simulink model "BattEv_Simscape"  (R2023a)
settings: Solver=ode23t  StartTime=0  StopTime=inf  RelTol=1e-3  EnableMultiTasking=on
model workspace (MAT data in the model file):
  Active_Scenario_Index = 1
  BattCurrent = [0 0.1 0.2 0.3 0.4 0.5 0.6 0.7 0.8 0.9 1 1.1 ... (49482 elements, 24741x2)]
  BattSocInit = 0.75
  BattTempInit = 25
  Battery : object (value not decoded)
  CellType = 1
  EV_current = 200
  EV_motion = [20 4 0.8]
  EV_sf = 2000
  Fs = 0
  Fv = 0.0025
  Jcomp = 0.0227
  Ki = 251.3274
  Kisa = 346.6583
  Kp_d = 0.47149
  Kp_q = 0.52125
  Ksa = 85.4316
  Ksf = 1996.2651
  Ld = 0.0003752
  Ldq = [0.0003752 0.0004148]
  Lq = 0.0004148
  Mechanical = [0.0227 0.0025 0]
  Np_Module = 31
  Ns_Module = 24
  NumModules = 4
  OverCellVoltageLimit = 4.19999980927
  P = 4
  PolePairs = 4
  R_bleed = 20
  Rs = 0.2
  T_eff_bp = [0 32.1428571429 64.2857142857 96.4285714286 128.571428571 160.714285714 192.857142857 225 257.142857143 289.285714286 321.428571429 353.571428571 ... (15 elements, 1x15)]
  T_env = 30
  T_init = 303.15
  T_max = 450
  T_mtpa = [0 13.3131834767 26.6278836885 39.9456159322 53.2678926341 66.5962219318 79.9321062746 93.277041051 106.632513247 120.000000141]
  T_set = 20.5
  Tc = 0.02
  TempInit = 288.15
  TestCase = 1
  UnderCellVoltageLimit = 2.5
  ba = 3.4029
  cell_area = 0.101908
  efficiency_table = [86.7 86.7 86.7 86.7 86.7 86.7 86.7 86.7 86.7 86.7 86.7 86.7 ... (180 elements, 12x15)]
  h_conv = 5
  id_mtpa = [0 -0.114523352646 -0.457989076459 -1.03008464374 -1.83029075221 -2.85788367342 -4.11193850568 -5.59133329791 -7.29475400168 -9.22070020138]
  idq0 = [0 0]
  idq_limits = [-9.220699542 166.993501392 167.247872355]
  iq_mtpa = [0 18.5827440345 37.1633719111 55.7397734896 74.3098506185 92.871523015 111.422734008 129.961456105 148.485696337 166.993501356]
  lambda_pm = 0.1194
  losses_table = [0 0 0 0 0 0 0 0 0 0 0 0 ... (180 elements, 12x15)]
  mdot_rev = 0.01
  mechanical = [0.0227 0.0025 0]
  omega_init = 0
  pipe : object (value not decoded)
  power_max = 211000
  pump : object (value not decoded)
  radiator : object (value not decoded)
  t_sim = 2474
  tank : object (value not decoded)
  theta_init = 0
  torque_max = 450
  ts = 0.1
  valve : object (value not decoded)
  w_eff_bp = [0 1600 3200 4477.56 4800 6400 8000 9600 11200 12800 14400 16000]
libraries: autolibpowerinfoutils x10, fl_lib x7, nesl_utility_internal x6, ee_lib x1
(part 2 of 2)

== system BattEv_Simscape/Battery Power Accounting ==
  BattV : Inport
  BattCurr : Inport  Port=2
  Bus Creator : BusCreator  Inputs=1
  Bus Creator1 : BusCreator  Inputs=1
  Gain : Gain  Gain=-1
  Gain1 : Gain
  Power Accounting : autolibpowerinfoutils/Power Accounting Bus Creator  AssctBlkSelPopup=Parent  RefBlkName='autolibsharedcoupling/Torsional Compliance'  PwrTrnsfrdCheckBox=on  PwrNotTrnsfrdCheckBox=on  PwrStoredCheckBox=off  aMode=aMode
  Product3 : Product
  Terminator2 : Terminator
  wires:
  Bus Creator/1 -> Power Accounting/1  "PwrTranfred"
  Gain/1 -> Bus Creator/1  "Batttransferred"
  Power Accounting/1 -> Terminator2/1
  Gain1/1 -> Bus Creator1/1  "BattNotTransferd"
  BattV/1 -> Product3/1
  BattCurr/1 -> Product3/2
  Bus Creator1/1 -> Power Accounting/2  "PwrNotTranfred"
  Product3/1 -> Gain1/1, Gain/1  "BattPwr"

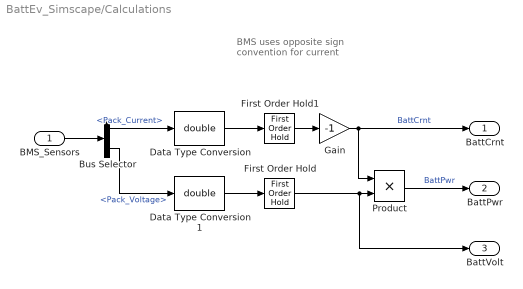
== system BattEv_Simscape/Calculations ==
  note: BMS uses opposite
      | sign convention for
      | current
  BMS_Sensors : Inport
  Bus Selector : BusSelector  OutputSignals=Pack_Current,Pack_Voltage
  Data Type Conversion : DataTypeConversion  OutDataTypeStr=double  SaturateOnIntegerOverflow=off  RndMeth=Floor
  Data Type Conversion1 : DataTypeConversion  OutDataTypeStr=double  SaturateOnIntegerOverflow=off  RndMeth=Floor
  First Order Hold : FirstOrderHold  ErrorTolerance=inf  AllowContinuousInput=on
  First Order Hold1 : FirstOrderHold  ErrorTolerance=inf  AllowContinuousInput=on
  Gain : Gain  Gain=-1
  Product : Product
  BattCrnt : Outport
  BattPwr : Outport  Port=2
  BattVolt : Outport  Port=3
  wires:
  Gain/1 -> BattCrnt/1, Product/1  "BattCrnt"
  BMS_Sensors/1 -> Bus Selector/1
  Data Type Conversion/1 -> First Order Hold1/1
  First Order Hold/1 -> BattVolt/1, Product/2
  First Order Hold1/1 -> Gain/1
  Bus Selector/1 -> Data Type Conversion/1  "<Pack_Current>"
  Bus Selector/2 -> Data Type Conversion1/1  "<Pack_Voltage>"
  Data Type Conversion1/1 -> First Order Hold/1
  Product/1 -> BattPwr/1  "BattPwr"

== system BattEv_Simscape/Cooling System ==
  BMS_Sensors : Inport
  AmbTmp : Inport  Port=2
  VehSpd : Inport  Port=3
  "Simscape " : Subsystem  VariantControl=1  ReferencedSubsystem=sscfluids_ev_battery_cooling_variant
      settings: PortSchema="{\"entries\":[{\"content\":{\"sides\":[{\"content\":{\"connectorIds\":[\"In1\",\"LConn1\",\"LConn2\",\"LConn3\",\"LConn4\",\"In3\",\"In2\"]},\"type\":\"ConnectorPlacement.EquallySpacedRectSide\",\"uuid\":\"91345e43-9326-4851-ae22-0115818e13bd\"},{\"content\":{\"connectorIds\":[\"RConn1\"],\"side\":\"RIGHT\"},\"type\":\"ConnectorPlacement.EquallySpacedRectSide\",\"uuid\":\"8fdec940-c4a1-4379-aa74-e54f16fb1812\"},{\"content\":{\"side\":\"TOP\"},\"type\":\"ConnectorPlacement.EquallySpacedRectSide\",\"uuid\":\"514fe1d2-faac-427c-8664-9f81e8916636\"}]},\"type\":\"ConnectorPlacement.EquallySpacedConnector\",\"uuid\":\"a4d1e3fd-26b0-4676-91d7-dc7f8f7b5942\"}],\"packageUris\":[\"http://schema.mathworks.com/mf0/Connector/R2020b\"],\"version\":\"1.0\"}"
  Pack 4 : PMIOPort  Side=Left
  Pack 3 : PMIOPort  Port=2  Side=Left
  Pack 2 : PMIOPort  Port=3  Side=Left
  Pack 1 : PMIOPort  Port=4  Side=Left
  Mot_H : PMIOPort  Port=5  Side=Right

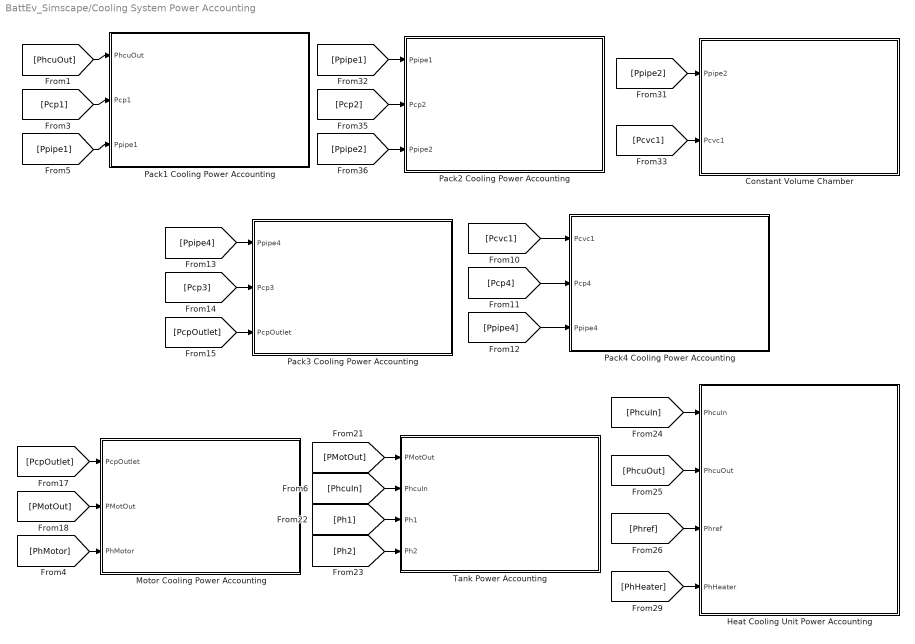
== system BattEv_Simscape/Cooling System Power Accounting ==
  Constant Volume Chamber : Subsystem
  Heat Cooling Unit Power Accounting : Subsystem
  Motor Cooling Power Accounting : Subsystem
  Pack1 Cooling Power Accounting : Subsystem
  Pack2 Cooling Power Accounting : Subsystem
  Pack3 Cooling Power Accounting : Subsystem
  Pack4 Cooling Power Accounting : Subsystem
  Tank Power Accounting : Subsystem
  wires:
  [Ph2] -> Tank Power Accounting/4(Ph2)
  [Ppipe2] -> Pack2 Cooling Power Accounting/3(Ppipe2)
  [Pcp2] -> Pack2 Cooling Power Accounting/2(Pcp2)
  [Phref] -> Heat Cooling Unit Power Accounting/3(Phref)
  [PMotOut] -> Motor Cooling Power Accounting/2(PMotOut)
  [PhcuIn] -> Tank Power Accounting/2(PhcuIn)
  [PcpOutlet] -> Motor Cooling Power Accounting/1(PcpOutlet)
  [PhcuIn] -> Heat Cooling Unit Power Accounting/1(PhcuIn)
  [PhcuOut] -> Pack1 Cooling Power Accounting/1(PhcuOut)
  [PhcuOut] -> Heat Cooling Unit Power Accounting/2(PhcuOut)
  [PcpOutlet] -> Pack3 Cooling Power Accounting/3(PcpOutlet)
  [Ppipe1] -> Pack1 Cooling Power Accounting/3(Ppipe1)
  [Pcp1] -> Pack1 Cooling Power Accounting/2(Pcp1)
  [Pcp3] -> Pack3 Cooling Power Accounting/2(Pcp3)
  [Pcvc1] -> Constant Volume Chamber/2(Pcvc1)
  [Ppipe4] -> Pack3 Cooling Power Accounting/1(Ppipe4)
  [Pcvc1] -> Pack4 Cooling Power Accounting/1(Pcvc1)
  [Ppipe1] -> Pack2 Cooling Power Accounting/1(Ppipe1)
  [Ppipe4] -> Pack4 Cooling Power Accounting/3(Ppipe4)
  [Ph1] -> Tank Power Accounting/3(Ph1)
  [PhMotor] -> Motor Cooling Power Accounting/3(PhMotor)
  [Ppipe2] -> Constant Volume Chamber/1(Ppipe2)
  [PMotOut] -> Tank Power Accounting/1(PMotOut)
  [PhHeater] -> Heat Cooling Unit Power Accounting/4(PhHeater)
  [Pcp4] -> Pack4 Cooling Power Accounting/2(Pcp4)

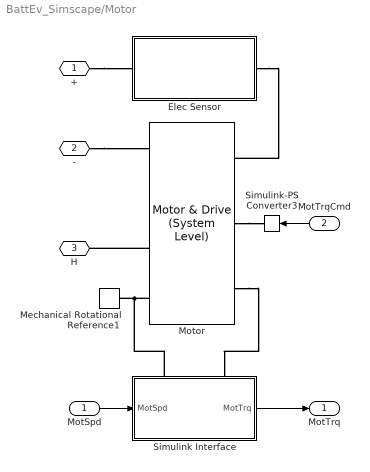
== system BattEv_Simscape/Motor ==
  MotSpd : Inport
  MotTrqCmd : Inport  Port=2
  Elec Sensor : Subsystem
  Mechanical Rotational Reference1 : fl_lib/Mechanical/Rotational Elements/Mechanical Rotational Reference
  Motor : ee_lib/Electromechanical/Motor & Drive (System Level)  torque_speed_param=ee.enum.electromech.envelope.torque_power  overtorque_param=ee.enum.electromech.overtorque.no  T_t=torque_max N*m  T_t_intermittent=[.36, .32, .28, 0] N*m  T_t_2D=[.09, .09, .09; .08, .08, .08; .07, .07, .07; 0, 0, 0] N*m  T_t_intermittent_2D=[.36, .36, .36; .32, .32, .32; .28, .28, .28; 0, 0, 0] N*m  w_t=Mot.w_eff_bp_EV_rear rpm  vdc_t=[6, 12, 24] V  torque_max=torque_max N*m  power_max=power_max W  torque_max_intermittent=0.4 N*m  power_max_intermittent=120 W  time_overtorque=30 s  time_recover=60 s  Tc=Tc s  losses_param=3  eff=100  w_eff=3750 rpm  T_eff=0.08 N*m  Piron=0 W  Pbase=0 W  w_eff_vec=w_eff_bp.*pi/30 rad/s  T_eff_vec=T_eff_bp N*m  v_eff_vec=[100, 250, 400] V  losses_mat=[1.49, 1.67, 2.21, 3.1; .42, .69, 1.14, 2.03; .06, .24, .78, 1.68; .42, .69, 1.14, 2.03; 1.49, 1.67, 2.21, 3.1] W  efficiency_mat=efficiency_table  losses_mat_3D=ones(5, 4, 3) W  efficiency_mat_3D=95 * ones(5, 4, 3)  Res=0 %Mot.supplyRes Ohm  enable_fault=simscape.enum.onoff.off  fault_condition=1  fault_threshold=0.5  J=5e-6 %Mot.inertia kg*m^2  lam=0 %Mot.damping N*m/(rad/s)  speed0=0 rpm  faulted_specify=off  faulted_priority=None  faulted=0  faulted_nominal_specify=off  faulted_nominal_unit=1  faulted_nominal_value=1  torqueLimitContinuous_specify=off  torqueLimitContinuous_priority=None  torqueLimitContinuous=0 N*m  torqueLimitContinuous_nominal_specify=off  torqueLimitContinuous_nominal_unit=N*m  torqueLimitContinuous_nominal_value=1  alpha=3.93e-3 1/K  Tmeas=25 degC  Tmeas2=125 degC  losses_mat_T2=[1.49, 1.74, 2.49, 3.74; .42, .67, 1.42, 2.67; .06, .31, 1.06, 2.31; .42, .67, 1.42, 2.67; 1.49, 1.74, 2.49, 3.74] W  efficiency_mat_T2=efficiency_table  losses_mat_3D_T2=ones(5, 4, 3) W  efficiency_mat_3D_T2=95 * ones(5, 4, 3)  thermal_mass=800 %Mot.thermalMass J/K  initial_temperature=300 K
      settings: InternalSimscapePortConfiguration="{\"Bottom\":[],\"Left\":[{\"id\":\"Vp\",\"label\":\"+\",\"type\":\"foundation.electrical.electrical\"},{\"id\":\"Tr\",\"label\":\"Tr\",\"type\":\"input\"},{\"id\":\"R\",\"label\":\"R\",\"type\":\"foundation.mechanical.rotational.rotational\"}],\"Right\":[{\"id\":\"Vm\",\"label\":\"-\",\"type\":\"foundation.electrical.electrical\"},{\"id\":\"Omega\",\"label\":\"w\",\"type\":\"output\"},{\"id\":\"H\",\"label\":\"H\",\"type\":\"foundation.thermal.thermal\"},{\"id\":\"C\",\"label\":\"C\",\"type\":\"foundation.mechanical.rotational.rotational\"}],\"Top\":[]}"
  Simulink Interface : Subsystem
      settings: PortSchema="{\"entries\":[{\"content\":{\"sides\":[{\"content\":{\"connectorIds\":[\"In1\"]},\"type\":\"ConnectorPlacement.EquallySpacedRectSide\",\"uuid\":\"bf4125d2-d804-43ee-b309-19af55b24a20\"},{\"content\":{\"connectorIds\":[\"Out1\"],\"side\":\"RIGHT\"},\"type\":\"ConnectorPlacement.EquallySpacedRectSide\",\"uuid\":\"b387e632-ddea-4493-9ae8-5e997efec9a6\"},{\"content\":{\"connectorIds\":[\"LConn1\",\"LConn2\"],\"side\":\"TOP\"},\"type\":\"ConnectorPlacement.EquallySpacedRectSide\",\"uuid\":\"41fd5ea6-0488-466e-8be0-697a42498d14\"}]},\"type\":\"ConnectorPlacement.EquallySpacedConnector\",\"uuid\":\"25cf6a75-933f-4ef5-8c77-b93f7c2ffe1f\"}],\"packageUris\":[\"http://schema.mathworks.com/mf0/Connector/R2020b\"],\"version\":\"1.0\"}"
  Simulink-PS Converter3 : nesl_utility_internal/Simulink-PS Converter  PhysicalDomain=network_engine_domain  SubClassName=ps_input  LeftPortType=input  RightPortType=output  PseudoPeriodic=off  Frequencies=[]  NoiseDistribution=none  NoiseParameters=[]  Unit=N*m  AffineConversion=off  FilteringAndDerivatives=provide  SimscapeFilterOrder=1  InputFilterTimeConstant=0.001  UdotUserProvided=0
  + : PMIOPort  Side=Left
  - : PMIOPort  Port=2  Side=Left
  H : PMIOPort  Port=3  Side=Left
  MotTrq : Outport  VectorParamsAs1DForOutWhenUnconnected=off
  wires:
  MotSpd/1 -> Simulink Interface/1(MotSpd)
  Simulink Interface/1(MotTrq) -> MotTrq/1
  MotTrqCmd/1 -> Simulink-PS Converter3/1
  connections:
  -/RConn1 -- Motor/RConn1
  Simulink Interface/LConn1 -- Motor/RConn4 -- Mechanical Rotational Reference1/LConn1
  Motor/LConn2 -- Simulink-PS Converter3/RConn1
  Motor/LConn3 -- Simulink Interface/LConn2
  +/RConn1 -- Elec Sensor/LConn1
  Elec Sensor/RConn1 -- Motor/LConn1
  Motor/RConn3 -- H/RConn1

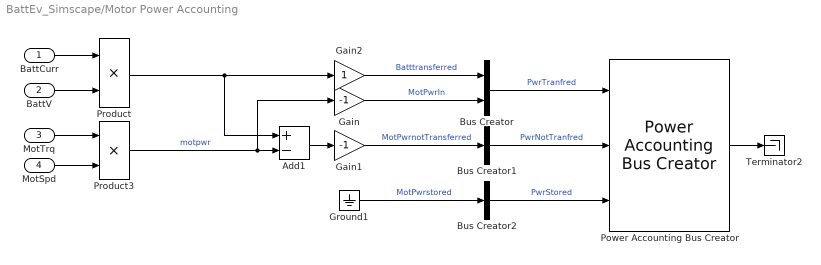
== system BattEv_Simscape/Motor Power Accounting ==
  BattCurr : Inport
  BattV : Inport  Port=2
  MotTrq : Inport  Port=3
  MotSpd : Inport  Port=4
  Add1 : Sum  Inputs=+-
  Bus Creator : BusCreator  Inputs=2
  Bus Creator1 : BusCreator  Inputs=1
  Bus Creator2 : BusCreator  Inputs=1
  Gain : Gain  Gain=-1
  Gain1 : Gain  Gain=-1
  Gain2 : Gain
  Ground1 : Ground
  Power Accounting Bus Creator : autolibpowerinfoutils/Power Accounting Bus Creator  AssctBlkSelPopup=Parent  RefBlkName='autolibsharedcoupling/Torsional Compliance'  PwrTrnsfrdCheckBox=on  PwrNotTrnsfrdCheckBox=on  PwrStoredCheckBox=on  aMode=aMode
  Product : Product
  Product3 : Product
  Terminator2 : Terminator
  wires:
  Gain2/1 -> Bus Creator/1  "Batttransferred"
  Product/1 -> Add1/1, Gain2/1
  BattV/1 -> Product/2
  BattCurr/1 -> Product/1
  Bus Creator/1 -> Power Accounting Bus Creator/1  "PwrTranfred"
  Gain/1 -> Bus Creator/2  "MotPwrIn"
  Power Accounting Bus Creator/1 -> Terminator2/1
  Ground1/1 -> Bus Creator2/1  "MotPwrstored"
  MotTrq/1 -> Product3/1
  MotSpd/1 -> Product3/2
  Bus Creator1/1 -> Power Accounting Bus Creator/2  "PwrNotTranfred"
  Bus Creator2/1 -> Power Accounting Bus Creator/3  "PwrStored"
  Product3/1 -> Gain/1, Add1/2  "motpwr"
  Gain1/1 -> Bus Creator1/1  "MotPwrnotTransferred"
  Add1/1 -> Gain1/1

== system BattEv_Simscape/Subsystem2 ==
  In Bus Element : Inport  PortName=BMS_Info  Element=SOC
  Bus Selector : BusSelector  OutputSignals=SOC_CC
  Data Type Conversion : DataTypeConversion  SaturateOnIntegerOverflow=off  RndMeth=Floor
  Rate Transition : RateTransition  Commented=through
  convert2percent : Gain  Gain=100
  BattSOC : Outport
  wires:
  In Bus Element/1 -> Bus Selector/1
  convert2percent/1 -> Data Type Conversion/1
  Bus Selector/1 -> convert2percent/1  "<SOC_CC>"
  Data Type Conversion/1 -> Rate Transition/1
  Rate Transition/1 -> BattSOC/1

== system BattEv_Simscape/Cooling System Power Accounting/Constant Volume Chamber ==
  Ppipe2 : Inport
  Pcvc1 : Inport  Port=2
  " Power Accounting" : autolibpowerinfoutils/Power Accounting Bus Creator  AssctBlkSelPopup=Parent  RefBlkName='autolibsharedcoupling/Torsional Compliance'  PwrTrnsfrdCheckBox=on  PwrNotTrnsfrdCheckBox=on  PwrStoredCheckBox=off  aMode=aMode
  Add : Sum  Inputs=+-
  Bus Creator : BusCreator  Inputs=2
  Bus Creator1 : BusCreator  Inputs=1
  Gain : Gain  Gain=-1
  Gain1 : Gain  Gain=-1
  Terminator2 : Terminator
  wires:
  Ppipe2/1 -> Bus Creator/1, Add/1  "Ppipe2"
  Gain/1 -> Bus Creator/2  "Pcvc1"
  Bus Creator/1 -> " Power Accounting"/1  "PwrTranfred"
  Pcvc1/1 -> Add/2, Gain/1
  Gain1/1 -> Bus Creator1/1  "PwrNotTrnsfrd"
  Bus Creator1/1 -> " Power Accounting"/2  "PwrNotTranfred"
  " Power Accounting"/1 -> Terminator2/1
  Add/1 -> Gain1/1

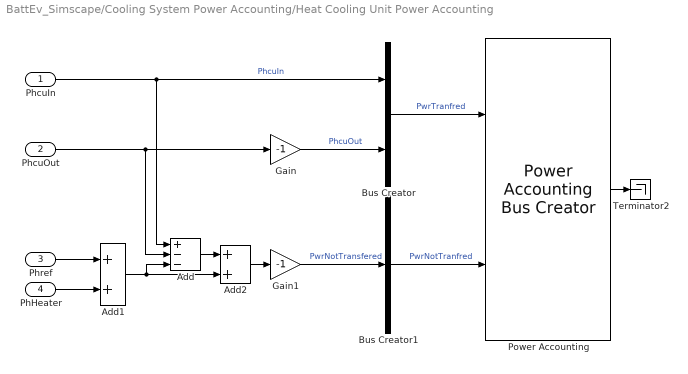
== system BattEv_Simscape/Cooling System Power Accounting/Heat Cooling Unit Power Accounting ==
  PhcuIn : Inport
  PhcuOut : Inport  Port=2
  Phref : Inport  Port=3
  PhHeater : Inport  Port=4
  Add : Sum  Inputs=+--
  Add1 : Sum
  Add2 : Sum
  Bus Creator : BusCreator  Inputs=2
  Bus Creator1 : BusCreator  Inputs=1
  Gain : Gain  Gain=-1
  Gain1 : Gain  Gain=-1
  Power Accounting : autolibpowerinfoutils/Power Accounting Bus Creator  AssctBlkSelPopup=Parent  RefBlkName='autolibsharedcoupling/Torsional Compliance'  PwrTrnsfrdCheckBox=on  PwrNotTrnsfrdCheckBox=on  PwrStoredCheckBox=off  aMode=aMode
  Terminator2 : Terminator
  wires:
  PhcuOut/1 -> Add/2, Gain/1
  Add2/1 -> Gain1/1
  Power Accounting/1 -> Terminator2/1
  Bus Creator1/1 -> Power Accounting/2  "PwrNotTranfred"
  Phref/1 -> Add1/1
  Gain1/1 -> Bus Creator1/1  "PwrNotTransfered"
  Bus Creator/1 -> Power Accounting/1  "PwrTranfred"
  Gain/1 -> Bus Creator/2  "PhcuOut"
  PhcuIn/1 -> Bus Creator/1, Add/1  "PhcuIn"
  PhHeater/1 -> Add1/2
  Add1/1 -> Add/3, Add2/2
  Add/1 -> Add2/1

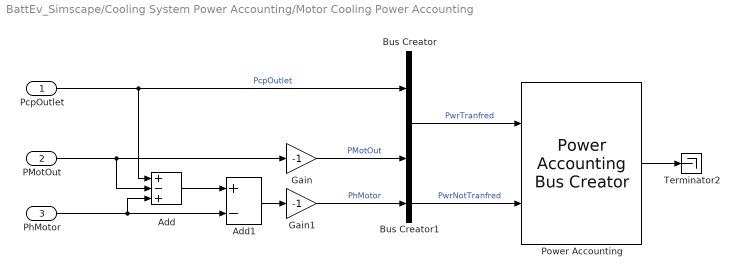
== system BattEv_Simscape/Cooling System Power Accounting/Motor Cooling Power Accounting ==
  PcpOutlet : Inport
  PMotOut : Inport  Port=2
  PhMotor : Inport  Port=3
  Add : Sum  Inputs=+-+
  Add1 : Sum  Inputs=+-
  Bus Creator : BusCreator  Inputs=2
  Bus Creator1 : BusCreator  Inputs=1
  Gain : Gain  Gain=-1
  Gain1 : Gain  Gain=-1
  Power Accounting : autolibpowerinfoutils/Power Accounting Bus Creator  AssctBlkSelPopup=Parent  RefBlkName='autolibsharedcoupling/Torsional Compliance'  PwrTrnsfrdCheckBox=on  PwrNotTrnsfrdCheckBox=on  PwrStoredCheckBox=off  aMode=aMode
  Terminator2 : Terminator
  wires:
  Add1/1 -> Gain1/1
  Power Accounting/1 -> Terminator2/1
  Bus Creator1/1 -> Power Accounting/2  "PwrNotTranfred"
  Add/1 -> Add1/1
  Gain1/1 -> Bus Creator1/1  "PhMotor"
  PMotOut/1 -> Gain/1, Add/2
  Bus Creator/1 -> Power Accounting/1  "PwrTranfred"
  Gain/1 -> Bus Creator/2  "PMotOut"
  PcpOutlet/1 -> Bus Creator/1, Add/1  "PcpOutlet"
  PhMotor/1 -> Add1/2, Add/3

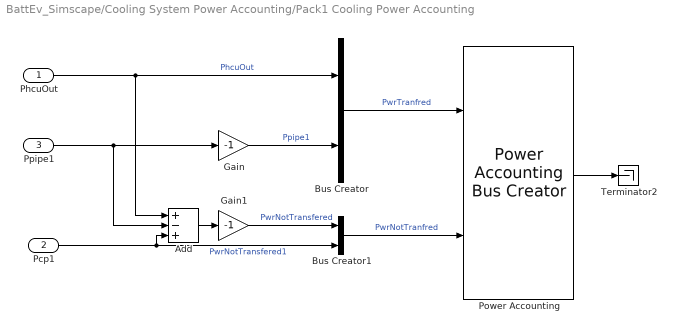
== system BattEv_Simscape/Cooling System Power Accounting/Pack1 Cooling Power Accounting ==
  PhcuOut : Inport
  Pcp1 : Inport  Port=2
  Ppipe1 : Inport  Port=3
  Add : Sum  Inputs=+-+
  Bus Creator : BusCreator  Inputs=2
  Bus Creator1 : BusCreator  Inputs=2
  Gain : Gain  Gain=-1
  Gain1 : Gain  Gain=-1
  Power Accounting : autolibpowerinfoutils/Power Accounting Bus Creator  AssctBlkSelPopup=Parent  RefBlkName='autolibsharedcoupling/Torsional Compliance'  PwrTrnsfrdCheckBox=on  PwrNotTrnsfrdCheckBox=on  PwrStoredCheckBox=off  aMode=aMode
  Terminator2 : Terminator
  wires:
  Add/1 -> Gain1/1
  Power Accounting/1 -> Terminator2/1
  Bus Creator1/1 -> Power Accounting/2  "PwrNotTranfred"
  Gain1/1 -> Bus Creator1/1  "PwrNotTransfered"
  Ppipe1/1 -> Gain/1, Add/2
  Bus Creator/1 -> Power Accounting/1  "PwrTranfred"
  Gain/1 -> Bus Creator/2  "Ppipe1"
  PhcuOut/1 -> Bus Creator/1, Add/1  "PhcuOut"
  Pcp1/1 -> Add/3, Bus Creator1/2  "PwrNotTransfered1"

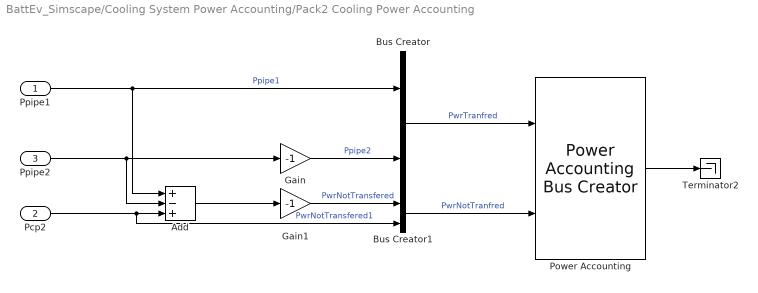
== system BattEv_Simscape/Cooling System Power Accounting/Pack2 Cooling Power Accounting ==
  Ppipe1 : Inport
  Pcp2 : Inport  Port=2
  Ppipe2 : Inport  Port=3
  Add : Sum  Inputs=+-+
  Bus Creator : BusCreator  Inputs=2
  Bus Creator1 : BusCreator  Inputs=2
  Gain : Gain  Gain=-1
  Gain1 : Gain  Gain=-1
  Power Accounting : autolibpowerinfoutils/Power Accounting Bus Creator  AssctBlkSelPopup=Parent  RefBlkName='autolibsharedcoupling/Torsional Compliance'  PwrTrnsfrdCheckBox=on  PwrNotTrnsfrdCheckBox=on  PwrStoredCheckBox=off  aMode=aMode
  Terminator2 : Terminator
  wires:
  Pcp2/1 -> Bus Creator1/2, Add/3  "PwrNotTransfered1"
  Ppipe1/1 -> Bus Creator/1, Add/1  "Ppipe1"
  Gain/1 -> Bus Creator/2  "Ppipe2"
  Bus Creator/1 -> Power Accounting/1  "PwrTranfred"
  Ppipe2/1 -> Add/2, Gain/1
  Gain1/1 -> Bus Creator1/1  "PwrNotTransfered"
  Bus Creator1/1 -> Power Accounting/2  "PwrNotTranfred"
  Power Accounting/1 -> Terminator2/1
  Add/1 -> Gain1/1

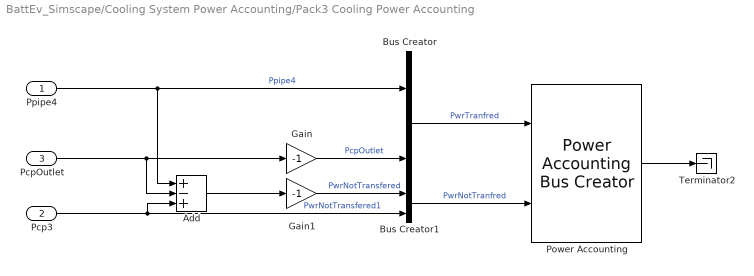
== system BattEv_Simscape/Cooling System Power Accounting/Pack3 Cooling Power Accounting ==
  Ppipe4 : Inport
  Pcp3 : Inport  Port=2
  PcpOutlet : Inport  Port=3
  Add : Sum  Inputs=+-+
  Bus Creator : BusCreator  Inputs=2
  Bus Creator1 : BusCreator  Inputs=2
  Gain : Gain  Gain=-1
  Gain1 : Gain  Gain=-1
  Power Accounting : autolibpowerinfoutils/Power Accounting Bus Creator  AssctBlkSelPopup=Parent  RefBlkName='autolibsharedcoupling/Torsional Compliance'  PwrTrnsfrdCheckBox=on  PwrNotTrnsfrdCheckBox=on  PwrStoredCheckBox=off  aMode=aMode
  Terminator2 : Terminator
  wires:
  Pcp3/1 -> Bus Creator1/2, Add/3  "PwrNotTransfered1"
  Ppipe4/1 -> Bus Creator/1, Add/1  "Ppipe4"
  Gain/1 -> Bus Creator/2  "PcpOutlet"
  Bus Creator/1 -> Power Accounting/1  "PwrTranfred"
  PcpOutlet/1 -> Add/2, Gain/1
  Gain1/1 -> Bus Creator1/1  "PwrNotTransfered"
  Bus Creator1/1 -> Power Accounting/2  "PwrNotTranfred"
  Power Accounting/1 -> Terminator2/1
  Add/1 -> Gain1/1

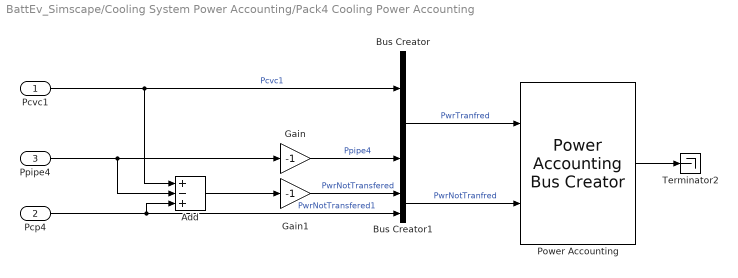
== system BattEv_Simscape/Cooling System Power Accounting/Pack4 Cooling Power Accounting ==
  Pcvc1 : Inport
  Pcp4 : Inport  Port=2
  Ppipe4 : Inport  Port=3
  Add : Sum  Inputs=+-+
  Bus Creator : BusCreator  Inputs=2
  Bus Creator1 : BusCreator  Inputs=2
  Gain : Gain  Gain=-1
  Gain1 : Gain  Gain=-1
  Power Accounting : autolibpowerinfoutils/Power Accounting Bus Creator  AssctBlkSelPopup=Parent  RefBlkName='autolibsharedcoupling/Torsional Compliance'  PwrTrnsfrdCheckBox=on  PwrNotTrnsfrdCheckBox=on  PwrStoredCheckBox=off  aMode=aMode
  Terminator2 : Terminator
  wires:
  Add/1 -> Gain1/1
  Power Accounting/1 -> Terminator2/1
  Bus Creator1/1 -> Power Accounting/2  "PwrNotTranfred"
  Gain1/1 -> Bus Creator1/1  "PwrNotTransfered"
  Ppipe4/1 -> Gain/1, Add/2
  Bus Creator/1 -> Power Accounting/1  "PwrTranfred"
  Gain/1 -> Bus Creator/2  "Ppipe4"
  Pcvc1/1 -> Bus Creator/1, Add/1  "Pcvc1"
  Pcp4/1 -> Add/3, Bus Creator1/2  "PwrNotTransfered1"

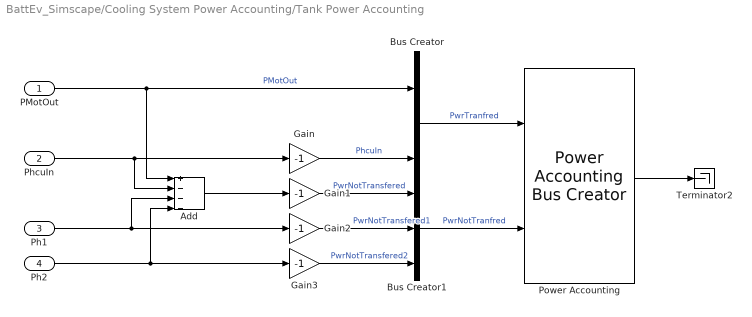
== system BattEv_Simscape/Cooling System Power Accounting/Tank Power Accounting ==
  PMotOut : Inport
  PhcuIn : Inport  Port=2
  Ph1 : Inport  Port=3
  Ph2 : Inport  Port=4
  Add : Sum  Inputs=+---
  Bus Creator : BusCreator  Inputs=2
  Bus Creator1 : BusCreator  Inputs=3
  Gain{,1..3} (4 alike) : Gain  Gain=-1
  Power Accounting : autolibpowerinfoutils/Power Accounting Bus Creator  AssctBlkSelPopup=Parent  RefBlkName='autolibsharedcoupling/Torsional Compliance'  PwrTrnsfrdCheckBox=on  PwrNotTrnsfrdCheckBox=on  PwrStoredCheckBox=off  aMode=aMode
  Terminator2 : Terminator
  wires:
  PMotOut/1 -> Bus Creator/1, Add/1  "PMotOut"
  Gain/1 -> Bus Creator/2  "PhcuIn"
  Bus Creator/1 -> Power Accounting/1  "PwrTranfred"
  Gain1/1 -> Bus Creator1/1  "PwrNotTransfered"
  Bus Creator1/1 -> Power Accounting/2  "PwrNotTranfred"
  Power Accounting/1 -> Terminator2/1
  Add/1 -> Gain1/1
  Ph2/1 -> Add/4, Gain3/1
  PhcuIn/1 -> Add/2, Gain/1
  Ph1/1 -> Add/3, Gain2/1
  Gain2/1 -> Bus Creator1/2  "PwrNotTransfered1"
  Gain3/1 -> Bus Creator1/3  "PwrNotTransfered2"

== system BattEv_Simscape/Motor/Elec Sensor ==
  Current Sensor2 : fl_lib/Electrical/Electrical Sensors/Current Sensor
  Electrical Reference : fl_lib/Electrical/Electrical Elements/Electrical Reference
  PS-Simulink Converter : nesl_utility_internal/PS-Simulink Converter  PhysicalDomain=network_engine_domain  SubClassName=ps_output  LeftPortType=input  RightPortType=output  PseudoPeriodic=off  Frequencies=[]  VectorFormat=1-D array  Unit=inherit  AffineConversion=off
  PS-Simulink Converter4 : nesl_utility_internal/PS-Simulink Converter  PhysicalDomain=network_engine_domain  SubClassName=ps_output  LeftPortType=input  RightPortType=output  PseudoPeriodic=off  Frequencies=[]  VectorFormat=1-D array  Unit=1  AffineConversion=off
  Product2 : Product
  Terminator : Terminator
  Voltage Sensor : fl_lib/Electrical/Electrical Sensors/Voltage Sensor
  + : PMIOPort  Side=Left
  - : PMIOPort  Port=2  Side=Right
  wires:
  PS-Simulink Converter4/1 -> Product2/2  "MotCurr"
  Product2/1 -> Terminator/1  "MotPwrElec"
  PS-Simulink Converter/1 -> Product2/1  "MotV"
  connections:
  Current Sensor2/RConn1 -- PS-Simulink Converter4/LConn1
  Current Sensor2/RConn2 -- -/RConn1
  +/RConn1 -- Voltage Sensor/LConn1 -- Current Sensor2/LConn1
  Electrical Reference/LConn1 -- Voltage Sensor/RConn2
  PS-Simulink Converter/LConn1 -- Voltage Sensor/RConn1

== system BattEv_Simscape/Motor/Simulink Interface ==
  MotSpd : Inport
  Ideal Angular Velocity Source1 : fl_lib/Mechanical/Mechanical Sources/Ideal Angular Velocity Source
  Ideal Torque Sensor1 : fl_lib/Mechanical/Mechanical Sensors/Ideal Torque Sensor
  Ideal Torque Sensor2 : fl_lib/Mechanical/Mechanical Sensors/Ideal Torque Sensor
  PS-Simulink Converter2 : nesl_utility_internal/PS-Simulink Converter  PhysicalDomain=network_engine_domain  SubClassName=ps_output  LeftPortType=input  RightPortType=output  PseudoPeriodic=off  Frequencies=[]  VectorFormat=1-D array  Unit=N*m  AffineConversion=off
  Simulink-PS Converter4 : nesl_utility_internal/Simulink-PS Converter  PhysicalDomain=network_engine_domain  SubClassName=ps_input  LeftPortType=input  RightPortType=output  PseudoPeriodic=off  Frequencies=[]  NoiseDistribution=none  NoiseParameters=[]  Unit=rad/s  AffineConversion=off  FilteringAndDerivatives=filter  SimscapeFilterOrder=1  InputFilterTimeConstant=0.001  UdotUserProvided=0
  C : PMIOPort  Side=Left
  R : PMIOPort  Port=2  Side=Left
  MotTrq : Outport
  wires:
  PS-Simulink Converter2/1 -> MotTrq/1  "MotTrq"
  MotSpd/1 -> Simulink-PS Converter4/1
  connections:
  Ideal Torque Sensor2/RConn2 -- PS-Simulink Converter2/LConn1
  Ideal Angular Velocity Source1/LConn1 -- Ideal Torque Sensor1/RConn1
  Simulink-PS Converter4/RConn1 -- Ideal Angular Velocity Source1/RConn1
  Ideal Torque Sensor2/RConn1 -- Ideal Torque Sensor1/LConn1
  Ideal Angular Velocity Source1/RConn2 -- C/RConn1
  R/RConn1 -- Ideal Torque Sensor2/LConn1
